simulink model "TorqueVect"  (R2022a)
settings: Solver=VariableStepAuto  StartTime=0.0  StopTime=300  RelTol=1e-3
PreLoadFcn:
  | run('Parameters\FSE_Parameters.m')
values from neighbouring files (symbols this model uses):
  Kd = 0;')    [open_carmaker_gui.m]
  Ki = 0    [open_carmaker_gui.m]
undefined symbols (not defined in the file or in its folder): BRegenEnabledButton, canChannel, CyalphaLookUp, efficiency, Fz_curve, Fz_scaling_long, gearR, izz, jw, kd, ki, Kp, kp, l_f, l_r, lambda, m, Mz_max, N, N_lat, N_long, P_max, pid_kd_lat, pid_kd_long, pid_ki_lat, pid_ki_long, pid_kp_lat, pid_kp_long, R_max, rw, steerR, T_i_max, TC_Decr_Gas, TC_Derivative, TC_Incr_Gas, TC_On, TC_Relay_Off, TC_Relay_On, tireCornerStiffness, Ts, TV_On, TV_Override, velocity_lookup, velocity_lookup_lat, y_ref, yrr_scaling
libraries: simulink x218, slpidlib x135, CarMaker4SL x73, TractionControlLibrary x13, canmsglib x9, canlib x8, TorqueVectoringLibrary x6, simulink_extras x4, PedalConversionLibrary x3, PowerControlLibrary x1
(part 10 of 26)

== system TorqueVect/CarMaker/IPG Vehicle/PowerTrain/PTControl Example/PTControl_PC_TC_MFE/New TC/TC R2 ==
  modified slip ratio reference : Inport
  lim 1 : Inport  Port=2
  modified slip ratio measurement : Inport  Port=3
  P_TC : Inport  Port=4
  D_TC : Inport  Port=5
  enable_tc : Inport  Port=6
  PID Controller : slpidlib/PID Controller  Commented=on  Controller=PD  Form=Parallel  TimeDomain=Discrete-time  UseExternalTs=off  SampleTime=-1  IntegratorMethod=Forward Euler  FilterMethod=Forward Euler  ControllerParametersSource=external  P=125  I=1  UseKiTs=on  D=0  N=100  UseFilter=on  TunerSelectOption=Transfer Function Based (PID Tuner App)  InitialConditionSource=internal  InitialConditionForIntegrator=0  InitialConditionForFilter=0  DifferentiatorICPrevScaledInput=0  ExternalReset=none  TrackingMode=off  Kt=1  LimitOutput=on  SatLimitsSource=external  UpperSaturationLimit=inf  LowerSaturationLimit=-inf  LinearizeAsGain=on  AntiWindupMode=clamping  Kb=1  POutMin=[]  POutMax=[]  IOutMin=[]  IOutMax=[]  DOutMin=[]  DOutMax=[]  NOutMin=[]  NOutMax=[]  SumOutMin=[]  SumOutMax=[]  SaturationOutMin=[]  SaturationOutMax=[]  PParamMin=[]  PParamMax=[]  IParamMin=[]  IParamMax=[]  DParamMin=[]  DParamMax=[]  NParamMin=[]  NParamMax=[]  KbParamMin=[]  KbParamMax=[]  KtParamMin=[]  KtParamMax=[]  KbOutMin=[]  KbOutMax=[]  KtOutMin=[]  KtOutMax=[]  IntegratorOutMin=[]  IntegratorOutMax=[]  FilterOutMin=[]  FilterOutMax=[]  SumI1OutMin=[]  SumI1OutMax=[]  SumI2OutMin=[]  SumI2OutMax=[]  SumI3OutMin=[]  SumI3OutMax=[]  SumI4OutMin=[]  SumI4OutMax=[]  SumDOutMin=[]  SumDOutMax=[]  DifferentiatorOutMin=[]  DifferentiatorOutMax=[]  FilterDiffOutCoefMin=[]  FilterDiffOutCoefMax=[]  ReciprocalOutMin=[]  ReciprocalOutMax=[]  SumDenOutMin=[]  SumDenOutMax=[]  SumNumOutMin=[]  SumNumOutMax=[]  DivideOutMin=[]  DivideOutMax=[]  UdiffTsProdOutMin=[]  UdiffTsProdOutMax=[]  NTsProdOutMin=[]  NTsProdOutMax=[]  UintegralTsProdOutMin=[]  UintegralTsProdOutMax=[]  UngainTsProdOutMin=[]  UngainTsProdOutMax=[]  ClampingZeroOutDataTypeStr=Inherit: Inherit via back propagation  ClampingZeroOutMin=[]  ClampingZeroOutMax=[]  FilterDenConstantOutDataTypeStr=Inherit: Inherit via back propagation  FilterDenConstantOutMin=[]  FilterDenConstantOutMax=[]  PCopyOutDataTypeStr=Inherit: Inherit via back propagation  PCopyOutMin=[]  PCopyOutMax=[]  NCopyOutDataTypeStr=Inherit: Inherit via back propagation  NCopyOutMin=[]  NCopyOutMax=[]  IntegratorContinuousStateAttributes=''  IntegratorStateMustResolveToSignalObject=off  IntegratorRTWStateStorageClass=Auto  FilterContinuousStateAttributes=''  FilterStateMustResolveToSignalObject=off  FilterRTWStateStorageClass=Auto  ParallelPVariant=ExternalParameters  IdealPVariant=Disabled  IVariant=Disabled  DVariant=ExternalParameters  IntegratorVariant=Disabled  SatVariant=External  AWVariant=Disabled  PCopyVariant=Disabled  TRVariant=Disabled  FdbkBlocksVariant=Forward  IdealPFdbkVariant=Disabled  SatFdbkVariant=Disabled  DerivativeFilterVariant=ForwardEulerFilter  NVariant=ExternalParameters  NCopyVariant=Disabled  FilterICVariant=InternalICsFilter  IntegratorICVariant=Disabled  ExternalResetVariant=Disabled  TRSumVariant=Passthrough  SumFdbkVariant=Disabled  SumVariant=Sum_PD  TsampFilterVariant=InternalTs  TsampNgainVariant=Passthrough  TsampIntegralVariant=Disabled_SignalSpec  ExternalSaturationOutDataTypeStr=Inherit: Same as second input  aMode=0
  Sum1 : Sum  Inputs=|-+
  Sum2 : Sum  Commented=on  Inputs=|-+
  traction_controller : Subsystem
  Control Effort 1 : Outport
  wires:
  modified slip ratio reference/1 -> Sum1/1
  modified slip ratio measurement/1 -> Sum1/2
  lim 1/1 -> Sum2/2, traction_controller/1(max_torque)
  PID Controller/1 -> Sum2/1
  traction_controller/1(delta_torque) -> Control Effort 1/1
  enable_tc/1 -> traction_controller/3(enable_tc)
  Sum1/1 -> traction_controller/2(dslip)
  P_TC/1 -> traction_controller/4(Kp)
  D_TC/1 -> traction_controller/5(Kd)

== system TorqueVect/CarMaker/IPG Vehicle/PowerTrain/PTControl Example/PTControl_PC_TC_MFE/New TC/TC R3 ==
  modified slip ratio reference : Inport
  lim 1 : Inport  Port=2
  modified slip ratio measurement : Inport  Port=3
  P_TC : Inport  Port=4
  D_TC : Inport  Port=5
  enable_tc : Inport  Port=6
  PID Controller : slpidlib/PID Controller  Commented=on  Controller=PD  Form=Parallel  TimeDomain=Discrete-time  UseExternalTs=off  SampleTime=-1  IntegratorMethod=Forward Euler  FilterMethod=Forward Euler  ControllerParametersSource=external  P=125  I=1  UseKiTs=on  D=0  N=100  UseFilter=on  TunerSelectOption=Transfer Function Based (PID Tuner App)  InitialConditionSource=internal  InitialConditionForIntegrator=0  InitialConditionForFilter=0  DifferentiatorICPrevScaledInput=0  ExternalReset=none  TrackingMode=off  Kt=1  LimitOutput=on  SatLimitsSource=external  UpperSaturationLimit=inf  LowerSaturationLimit=-inf  LinearizeAsGain=on  AntiWindupMode=clamping  Kb=1  POutMin=[]  POutMax=[]  IOutMin=[]  IOutMax=[]  DOutMin=[]  DOutMax=[]  NOutMin=[]  NOutMax=[]  SumOutMin=[]  SumOutMax=[]  SaturationOutMin=[]  SaturationOutMax=[]  PParamMin=[]  PParamMax=[]  IParamMin=[]  IParamMax=[]  DParamMin=[]  DParamMax=[]  NParamMin=[]  NParamMax=[]  KbParamMin=[]  KbParamMax=[]  KtParamMin=[]  KtParamMax=[]  KbOutMin=[]  KbOutMax=[]  KtOutMin=[]  KtOutMax=[]  IntegratorOutMin=[]  IntegratorOutMax=[]  FilterOutMin=[]  FilterOutMax=[]  SumI1OutMin=[]  SumI1OutMax=[]  SumI2OutMin=[]  SumI2OutMax=[]  SumI3OutMin=[]  SumI3OutMax=[]  SumI4OutMin=[]  SumI4OutMax=[]  SumDOutMin=[]  SumDOutMax=[]  DifferentiatorOutMin=[]  DifferentiatorOutMax=[]  FilterDiffOutCoefMin=[]  FilterDiffOutCoefMax=[]  ReciprocalOutMin=[]  ReciprocalOutMax=[]  SumDenOutMin=[]  SumDenOutMax=[]  SumNumOutMin=[]  SumNumOutMax=[]  DivideOutMin=[]  DivideOutMax=[]  UdiffTsProdOutMin=[]  UdiffTsProdOutMax=[]  NTsProdOutMin=[]  NTsProdOutMax=[]  UintegralTsProdOutMin=[]  UintegralTsProdOutMax=[]  UngainTsProdOutMin=[]  UngainTsProdOutMax=[]  ClampingZeroOutDataTypeStr=Inherit: Inherit via back propagation  ClampingZeroOutMin=[]  ClampingZeroOutMax=[]  FilterDenConstantOutDataTypeStr=Inherit: Inherit via back propagation  FilterDenConstantOutMin=[]  FilterDenConstantOutMax=[]  PCopyOutDataTypeStr=Inherit: Inherit via back propagation  PCopyOutMin=[]  PCopyOutMax=[]  NCopyOutDataTypeStr=Inherit: Inherit via back propagation  NCopyOutMin=[]  NCopyOutMax=[]  IntegratorContinuousStateAttributes=''  IntegratorStateMustResolveToSignalObject=off  IntegratorRTWStateStorageClass=Auto  FilterContinuousStateAttributes=''  FilterStateMustResolveToSignalObject=off  FilterRTWStateStorageClass=Auto  ParallelPVariant=ExternalParameters  IdealPVariant=Disabled  IVariant=Disabled  DVariant=ExternalParameters  IntegratorVariant=Disabled  SatVariant=External  AWVariant=Disabled  PCopyVariant=Disabled  TRVariant=Disabled  FdbkBlocksVariant=Forward  IdealPFdbkVariant=Disabled  SatFdbkVariant=Disabled  DerivativeFilterVariant=ForwardEulerFilter  NVariant=ExternalParameters  NCopyVariant=Disabled  FilterICVariant=InternalICsFilter  IntegratorICVariant=Disabled  ExternalResetVariant=Disabled  TRSumVariant=Passthrough  SumFdbkVariant=Disabled  SumVariant=Sum_PD  TsampFilterVariant=InternalTs  TsampNgainVariant=Passthrough  TsampIntegralVariant=Disabled_SignalSpec  ExternalSaturationOutDataTypeStr=Inherit: Same as second input  aMode=0
  Sum1 : Sum  Inputs=|-+
  Sum2 : Sum  Commented=on  Inputs=|-+
  traction_controller : Subsystem
  Control Effort 1 : Outport
  wires:
  modified slip ratio reference/1 -> Sum1/1
  modified slip ratio measurement/1 -> Sum1/2
  lim 1/1 -> Sum2/2, traction_controller/1(max_torque)
  PID Controller/1 -> Sum2/1
  traction_controller/1(delta_torque) -> Control Effort 1/1
  enable_tc/1 -> traction_controller/3(enable_tc)
  Sum1/1 -> traction_controller/2(dslip)
  P_TC/1 -> traction_controller/4(Kp)
  D_TC/1 -> traction_controller/5(Kd)

== system TorqueVect/CarMaker/IPG Vehicle/PowerTrain/PTControl Example/PTControl_PC_TC_MFE/New TC/TC R4 ==
  modified slip ratio reference : Inport
  lim 1 : Inport  Port=2
  modified slip ratio measurement : Inport  Port=3
  P_TC : Inport  Port=4
  D_TC : Inport  Port=5
  enable_tc : Inport  Port=6
  PID Controller : slpidlib/PID Controller  Commented=on  Controller=PD  Form=Parallel  TimeDomain=Discrete-time  UseExternalTs=off  SampleTime=-1  IntegratorMethod=Forward Euler  FilterMethod=Forward Euler  ControllerParametersSource=external  P=125  I=1  UseKiTs=on  D=0  N=100  UseFilter=on  TunerSelectOption=Transfer Function Based (PID Tuner App)  InitialConditionSource=internal  InitialConditionForIntegrator=0  InitialConditionForFilter=0  DifferentiatorICPrevScaledInput=0  ExternalReset=none  TrackingMode=off  Kt=1  LimitOutput=on  SatLimitsSource=external  UpperSaturationLimit=inf  LowerSaturationLimit=-inf  LinearizeAsGain=on  AntiWindupMode=clamping  Kb=1  POutMin=[]  POutMax=[]  IOutMin=[]  IOutMax=[]  DOutMin=[]  DOutMax=[]  NOutMin=[]  NOutMax=[]  SumOutMin=[]  SumOutMax=[]  SaturationOutMin=[]  SaturationOutMax=[]  PParamMin=[]  PParamMax=[]  IParamMin=[]  IParamMax=[]  DParamMin=[]  DParamMax=[]  NParamMin=[]  NParamMax=[]  KbParamMin=[]  KbParamMax=[]  KtParamMin=[]  KtParamMax=[]  KbOutMin=[]  KbOutMax=[]  KtOutMin=[]  KtOutMax=[]  IntegratorOutMin=[]  IntegratorOutMax=[]  FilterOutMin=[]  FilterOutMax=[]  SumI1OutMin=[]  SumI1OutMax=[]  SumI2OutMin=[]  SumI2OutMax=[]  SumI3OutMin=[]  SumI3OutMax=[]  SumI4OutMin=[]  SumI4OutMax=[]  SumDOutMin=[]  SumDOutMax=[]  DifferentiatorOutMin=[]  DifferentiatorOutMax=[]  FilterDiffOutCoefMin=[]  FilterDiffOutCoefMax=[]  ReciprocalOutMin=[]  ReciprocalOutMax=[]  SumDenOutMin=[]  SumDenOutMax=[]  SumNumOutMin=[]  SumNumOutMax=[]  DivideOutMin=[]  DivideOutMax=[]  UdiffTsProdOutMin=[]  UdiffTsProdOutMax=[]  NTsProdOutMin=[]  NTsProdOutMax=[]  UintegralTsProdOutMin=[]  UintegralTsProdOutMax=[]  UngainTsProdOutMin=[]  UngainTsProdOutMax=[]  ClampingZeroOutDataTypeStr=Inherit: Inherit via back propagation  ClampingZeroOutMin=[]  ClampingZeroOutMax=[]  FilterDenConstantOutDataTypeStr=Inherit: Inherit via back propagation  FilterDenConstantOutMin=[]  FilterDenConstantOutMax=[]  PCopyOutDataTypeStr=Inherit: Inherit via back propagation  PCopyOutMin=[]  PCopyOutMax=[]  NCopyOutDataTypeStr=Inherit: Inherit via back propagation  NCopyOutMin=[]  NCopyOutMax=[]  IntegratorContinuousStateAttributes=''  IntegratorStateMustResolveToSignalObject=off  IntegratorRTWStateStorageClass=Auto  FilterContinuousStateAttributes=''  FilterStateMustResolveToSignalObject=off  FilterRTWStateStorageClass=Auto  ParallelPVariant=ExternalParameters  IdealPVariant=Disabled  IVariant=Disabled  DVariant=ExternalParameters  IntegratorVariant=Disabled  SatVariant=External  AWVariant=Disabled  PCopyVariant=Disabled  TRVariant=Disabled  FdbkBlocksVariant=Forward  IdealPFdbkVariant=Disabled  SatFdbkVariant=Disabled  DerivativeFilterVariant=ForwardEulerFilter  NVariant=ExternalParameters  NCopyVariant=Disabled  FilterICVariant=InternalICsFilter  IntegratorICVariant=Disabled  ExternalResetVariant=Disabled  TRSumVariant=Passthrough  SumFdbkVariant=Disabled  SumVariant=Sum_PD  TsampFilterVariant=InternalTs  TsampNgainVariant=Passthrough  TsampIntegralVariant=Disabled_SignalSpec  ExternalSaturationOutDataTypeStr=Inherit: Same as second input  aMode=0
  Sum1 : Sum  Inputs=|-+
  Sum2 : Sum  Commented=on  Inputs=|-+
  traction_controller : Subsystem
  Control Effort 1 : Outport
  wires:
  modified slip ratio reference/1 -> Sum1/1
  modified slip ratio measurement/1 -> Sum1/2
  lim 1/1 -> Sum2/2, traction_controller/1(max_torque)
  PID Controller/1 -> Sum2/1
  traction_controller/1(delta_torque) -> Control Effort 1/1
  enable_tc/1 -> traction_controller/3(enable_tc)
  Sum1/1 -> traction_controller/2(dslip)
  P_TC/1 -> traction_controller/4(Kp)
  D_TC/1 -> traction_controller/5(Kd)

== system TorqueVect/CarMaker/IPG Vehicle/PowerTrain/PTControl Example/PTControl_PC_TC_MFE/Subsystem1/Subsystem ==
  rThrottlePedal : Inport
  vLong : Inport  Port=2
  BRegenEnabledButton : Inport  Port=3
  MMotorFL : Inport  Port=4
  MMotorFR : Inport  Port=5
  MMotorRL : Inport  Port=6
  MMotorRR : Inport  Port=7
  nMotorFL : Inport  Port=8
  nMotorFR : Inport  Port=9
  nMotorRL : Inport  Port=10
  nMotorRR : Inport  Port=11
  PMeasured : Inport  Port=12
  BMeasuredEnable : Inport  Port=13
  rSplitF : Inport  Port=14
  rRegenSplitF : Inport  Port=15
  PRegenLimit : Inport  Port=16
  PLimit : Inport  Port=17
  FF_PC : Inport  Port=18
  FF_RC : Inport  Port=19
  P_PC : Inport  Port=20
  D_PC : Inport  Port=21
  MMotorMax : Inport  Port=22
  Add{,1..3} (4 alike) : Sum  Inputs=-+
  PedalConversion : PedalConversionLibrary/PedalConversion  SystemSampleTime=-1  VariantActivationTime=update diagram  Latency=0  AutoFrameSizeCalculation=off
  PowerControl : PowerControlLibrary/PowerControl  SystemSampleTime=-1  VariantActivationTime=update diagram  Latency=0  AutoFrameSizeCalculation=off
  TorqueSplit : TorqueVectoringLibrary/TorqueSplit  SystemSampleTime=-1  VariantActivationTime=update diagram  Latency=0  AutoFrameSizeCalculation=off
  MMotorDemandFL : Outport
  MMotorDemandFR : Outport  Port=2
  MMotorDemandRL : Outport  Port=3
  MMotorDemandRR : Outport  Port=4
  wires:
  rThrottlePedal/1 -> [rThrottlePedal]
  [rThrottlePedal] -> PedalConversion/1
  [rThrottlePedal] -> PowerControl/13
  vLong/1 -> PedalConversion/3
  BRegenEnabledButton/1 -> PedalConversion/2
  MMotorFL/1 -> PowerControl/1
  MMotorFR/1 -> PowerControl/2
  MMotorRL/1 -> PowerControl/3
  MMotorRR/1 -> PowerControl/4
  nMotorFL/1 -> PowerControl/5
  nMotorFR/1 -> PowerControl/6
  nMotorRL/1 -> PowerControl/7
  nMotorRR/1 -> PowerControl/8
  PMeasured/1 -> PowerControl/9
  BMeasuredEnable/1 -> PowerControl/10
  PRegenLimit/1 -> PowerControl/15
  PLimit/1 -> PowerControl/16
  FF_PC/1 -> PowerControl/17
  FF_RC/1 -> PowerControl/18
  P_PC/1 -> PowerControl/19
  D_PC/1 -> PowerControl/20
  Add/1 -> MMotorDemandFL/1
  PowerControl/1 -> Add/1
  rSplitF/1 -> [rSplitF]
  [rSplitF] -> TorqueSplit/1
  rRegenSplitF/1 -> TorqueSplit/2
  PedalConversion/1 -> PowerControl/14, TorqueSplit/3
  MMotorMax/1 -> TorqueSplit/4
  [rSplitF] -> PowerControl/12
  PedalConversion/2 -> PowerControl/11
  TorqueSplit/1 -> [MMotorRequestFL]
  TorqueSplit/2 -> [MMotorRequestFR]
  TorqueSplit/3 -> [MMotorRequestRL]
  TorqueSplit/4 -> [MMotorRequestRR]
  [MMotorRequestFL] -> Add/2
  Add1/1 -> MMotorDemandFR/1
  PowerControl/2 -> Add1/1
  [MMotorRequestFR] -> Add1/2
  Add2/1 -> MMotorDemandRL/1
  PowerControl/3 -> Add2/1
  [MMotorRequestRL] -> Add2/2
  Add3/1 -> MMotorDemandRR/1
  PowerControl/4 -> Add3/1
  [MMotorRequestRR] -> Add3/2

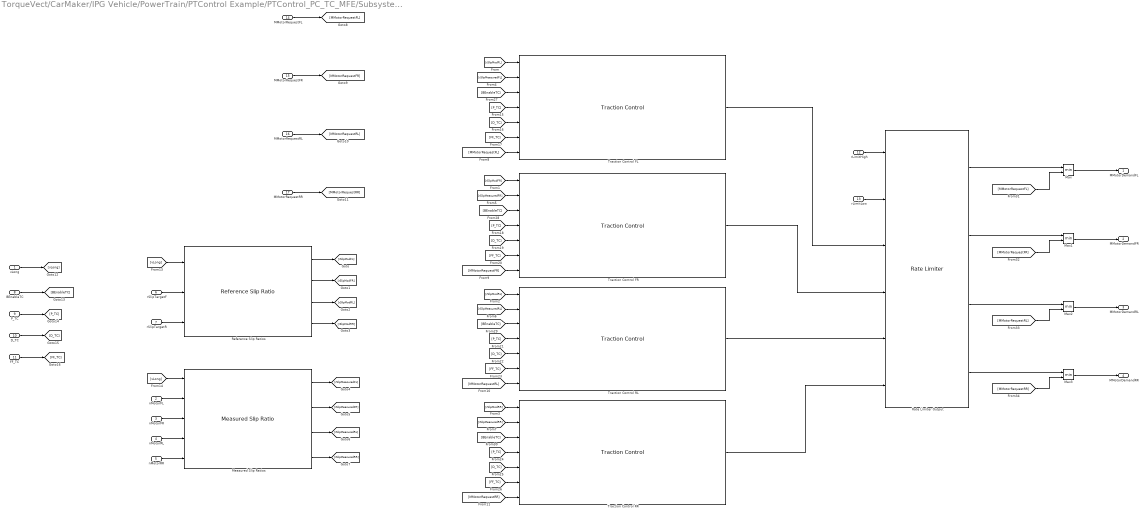
== system TorqueVect/CarMaker/IPG Vehicle/PowerTrain/PTControl Example/PTControl_PC_TC_MFE/Subsystem1/TC ==
  vLong : Inport
  nMotorFL : Inport  Port=2
  nMotorFR : Inport  Port=3
  nMotorRL : Inport  Port=4
  nMotorRR : Inport  Port=5
  rSlipTargetF : Inport  Port=6
  rSlipTargetR : Inport  Port=7
  BEnableTC : Inport  Port=8
  P_TC : Inport  Port=9
  D_TC : Inport  Port=10
  FF_TC : Inport  Port=11
  rLimitHigh : Inport  Port=12
  rLimitLow : Inport  Port=13
  MMotorRequestFL : Inport  Port=14
  MMotorRequestFR : Inport  Port=15
  MMotorRequestRL : Inport  Port=16
  MMotorRequestRR : Inport  Port=17
  Max{,1..3} (4 alike) : MinMax  Inputs=2
  Measured Slip Ratios : TractionControlLibrary/Measured Slip Ratio  SystemSampleTime=-1  VariantActivationTime=update diagram  Latency=0  AutoFrameSizeCalculation=off
  Rate Limiter Output : TractionControlLibrary/Rate Limiter  SystemSampleTime=-1  VariantActivationTime=update diagram  Latency=0  AutoFrameSizeCalculation=off
  Reference Slip Ratios : TractionControlLibrary/Reference Slip Ratio  SystemSampleTime=-1  VariantActivationTime=update diagram  Latency=0  AutoFrameSizeCalculation=off
  Traction Control FL : TractionControlLibrary/Traction Control  SystemSampleTime=-1  VariantActivationTime=update diagram  Latency=0  AutoFrameSizeCalculation=off
  Traction Control FR : TractionControlLibrary/Traction Control  SystemSampleTime=-1  VariantActivationTime=update diagram  Latency=0  AutoFrameSizeCalculation=off
  Traction Control RL : TractionControlLibrary/Traction Control  SystemSampleTime=-1  VariantActivationTime=update diagram  Latency=0  AutoFrameSizeCalculation=off
  Traction Control RR : TractionControlLibrary/Traction Control  SystemSampleTime=-1  VariantActivationTime=update diagram  Latency=0  AutoFrameSizeCalculation=off
  MMotorDemandFL : Outport
  MMotorDemandFR : Outport  Port=2
  MMotorDemandRL : Outport  Port=3
  MMotorDemandRR : Outport  Port=4
  wires:
  Traction Control FL/1 -> Rate Limiter Output/3
  Traction Control FR/1 -> Rate Limiter Output/4
  Traction Control RL/1 -> Rate Limiter Output/5
  Traction Control RR/1 -> Rate Limiter Output/6
  Reference Slip Ratios/1 -> [rSlipModFL]
  Reference Slip Ratios/2 -> [rSlipModFR]
  Reference Slip Ratios/3 -> [rSlipModRL]
  Reference Slip Ratios/4 -> [rSlipModRR]
  [rSlipModFL] -> Traction Control FL/1
  [rSlipModFR] -> Traction Control FR/1
  [rSlipModRL] -> Traction Control RL/1
  [rSlipModRR] -> Traction Control RR/1
  Measured Slip Ratios/1 -> [rSlipMeasuredFL]
  Measured Slip Ratios/2 -> [rSlipMeasuredFR]
  Measured Slip Ratios/3 -> [rSlipMeasuredRL]
  Measured Slip Ratios/4 -> [rSlipMeasuredRR]
  [rSlipMeasuredFL] -> Traction Control FL/2
  [rSlipMeasuredFR] -> Traction Control FR/2
  [rSlipMeasuredRL] -> Traction Control RL/2
  [rSlipMeasuredRR] -> Traction Control RR/2
  MMotorRequestFL/1 -> [MMotorRequestFL]
  MMotorRequestFR/1 -> [MMotorRequestFR]
  MMotorRequestRL/1 -> [MMotorRequestRL]
  MMotorRequestRR/1 -> [MMotorRequestRR]
  [MMotorRequestFL] -> Traction Control FL/7
  [MMotorRequestFR] -> Traction Control FR/7
  [MMotorRequestRL] -> Traction Control RL/7
  [MMotorRequestRR] -> Traction Control RR/7
  vLong/1 -> [vLong]
  [vLong] -> Reference Slip Ratios/1
  [vLong] -> Measured Slip Ratios/1
  nMotorFL/1 -> Measured Slip Ratios/2
  nMotorFR/1 -> Measured Slip Ratios/3
  nMotorRL/1 -> Measured Slip Ratios/4
  nMotorRR/1 -> Measured Slip Ratios/5
  rSlipTargetF/1 -> Reference Slip Ratios/2
  rSlipTargetR/1 -> Reference Slip Ratios/3
  BEnableTC/1 -> [BEnableTC]
  P_TC/1 -> [P_TC]
  D_TC/1 -> [D_TC]
  FF_TC/1 -> [FF_TC]
  [P_TC] -> Traction Control FL/4
  [D_TC] -> Traction Control FL/5
  [FF_TC] -> Traction Control FL/6
  [FF_TC] -> Traction Control FR/6
  [D_TC] -> Traction Control FR/5
  [P_TC] -> Traction Control FR/4
  [FF_TC] -> Traction Control RL/6
  [D_TC] -> Traction Control RL/5
  [P_TC] -> Traction Control RL/4
  [FF_TC] -> Traction Control RR/6
  [D_TC] -> Traction Control RR/5
  [P_TC] -> Traction Control RR/4
  [BEnableTC] -> Traction Control FL/3
  [BEnableTC] -> Traction Control FR/3
  [BEnableTC] -> Traction Control RL/3
  [BEnableTC] -> Traction Control RR/3
  rLimitHigh/1 -> Rate Limiter Output/1
  rLimitLow/1 -> Rate Limiter Output/2
  Rate Limiter Output/1 -> Max/1
  [MMotorRequestFL] -> Max/2
  Max/1 -> MMotorDemandFL/1
  Rate Limiter Output/2 -> Max1/1
  Max1/1 -> MMotorDemandFR/1
  [MMotorRequestFR] -> Max1/2
  Rate Limiter Output/3 -> Max2/1
  Max2/1 -> MMotorDemandRL/1
  [MMotorRequestRL] -> Max2/2
  Rate Limiter Output/4 -> Max3/1
  Max3/1 -> MMotorDemandRR/1
  [MMotorRequestRR] -> Max3/2

== system TorqueVect/CarMaker/IPG Vehicle/PowerTrain/PTControl Example/PTControl_TC_MFE/New TC/Reference Generator1 ==
  note: Modified slip ratio targets
  note: Vehicle velocity
  note: For throttle sign and Product:
      | If positive, normal reference
      | If negative (regen), similar reference but negative (negative target slip*times speed), this might need to change to account for regen limits
      | If 0, target zero
  x2 : Inport
  Front SR Target : Inport  Port=2
  Rear SR Target : Inport  Port=3
  Constant : Constant
  Product1 : Product
  Product2 : Product
  Switch : Switch  Criteria=u2 > Threshold  Threshold=1  SaturateOnIntegerOverflow=off  InputSameDT=off
  R1 : Outport
  L1 : Outport  Port=2
  R2 : Outport  Port=3
  L2 : Outport  Port=4
  wires:
  Front SR Target/1 -> Product1/1
  Product1/1 -> L1/1, R1/1
  Product2/1 -> L2/1, R2/1
  Rear SR Target/1 -> Product2/2
  Switch/1 -> Product2/1, Product1/2
  x2/1 -> Switch/1, Switch/2
  Constant/1 -> Switch/3

== system TorqueVect/CarMaker/IPG Vehicle/PowerTrain/PTControl Example/PTControl_TC_MFE/New TC/TC R1 ==
  modified slip ratio reference : Inport
  lim 1 : Inport  Port=2
  modified slip ratio measurement : Inport  Port=3
  P_TC : Inport  Port=4
  D_TC : Inport  Port=5
  enable_tc : Inport  Port=6
  PID Controller : slpidlib/PID Controller  Commented=on  Controller=PD  Form=Parallel  TimeDomain=Discrete-time  UseExternalTs=off  SampleTime=-1  IntegratorMethod=Forward Euler  FilterMethod=Forward Euler  ControllerParametersSource=external  P=125  I=1  UseKiTs=on  D=0  N=100  UseFilter=on  TunerSelectOption=Transfer Function Based (PID Tuner App)  InitialConditionSource=internal  InitialConditionForIntegrator=0  InitialConditionForFilter=0  DifferentiatorICPrevScaledInput=0  ExternalReset=none  TrackingMode=off  Kt=1  LimitOutput=on  SatLimitsSource=external  UpperSaturationLimit=inf  LowerSaturationLimit=-inf  LinearizeAsGain=on  AntiWindupMode=clamping  Kb=1  POutMin=[]  POutMax=[]  IOutMin=[]  IOutMax=[]  DOutMin=[]  DOutMax=[]  NOutMin=[]  NOutMax=[]  SumOutMin=[]  SumOutMax=[]  SaturationOutMin=[]  SaturationOutMax=[]  PParamMin=[]  PParamMax=[]  IParamMin=[]  IParamMax=[]  DParamMin=[]  DParamMax=[]  NParamMin=[]  NParamMax=[]  KbParamMin=[]  KbParamMax=[]  KtParamMin=[]  KtParamMax=[]  KbOutMin=[]  KbOutMax=[]  KtOutMin=[]  KtOutMax=[]  IntegratorOutMin=[]  IntegratorOutMax=[]  FilterOutMin=[]  FilterOutMax=[]  SumI1OutMin=[]  SumI1OutMax=[]  SumI2OutMin=[]  SumI2OutMax=[]  SumI3OutMin=[]  SumI3OutMax=[]  SumI4OutMin=[]  SumI4OutMax=[]  SumDOutMin=[]  SumDOutMax=[]  DifferentiatorOutMin=[]  DifferentiatorOutMax=[]  FilterDiffOutCoefMin=[]  FilterDiffOutCoefMax=[]  ReciprocalOutMin=[]  ReciprocalOutMax=[]  SumDenOutMin=[]  SumDenOutMax=[]  SumNumOutMin=[]  SumNumOutMax=[]  DivideOutMin=[]  DivideOutMax=[]  UdiffTsProdOutMin=[]  UdiffTsProdOutMax=[]  NTsProdOutMin=[]  NTsProdOutMax=[]  UintegralTsProdOutMin=[]  UintegralTsProdOutMax=[]  UngainTsProdOutMin=[]  UngainTsProdOutMax=[]  ClampingZeroOutDataTypeStr=Inherit: Inherit via back propagation  ClampingZeroOutMin=[]  ClampingZeroOutMax=[]  FilterDenConstantOutDataTypeStr=Inherit: Inherit via back propagation  FilterDenConstantOutMin=[]  FilterDenConstantOutMax=[]  PCopyOutDataTypeStr=Inherit: Inherit via back propagation  PCopyOutMin=[]  PCopyOutMax=[]  NCopyOutDataTypeStr=Inherit: Inherit via back propagation  NCopyOutMin=[]  NCopyOutMax=[]  IntegratorContinuousStateAttributes=''  IntegratorStateMustResolveToSignalObject=off  IntegratorRTWStateStorageClass=Auto  FilterContinuousStateAttributes=''  FilterStateMustResolveToSignalObject=off  FilterRTWStateStorageClass=Auto  ParallelPVariant=ExternalParameters  IdealPVariant=Disabled  IVariant=Disabled  DVariant=ExternalParameters  IntegratorVariant=Disabled  SatVariant=External  AWVariant=Disabled  PCopyVariant=Disabled  TRVariant=Disabled  FdbkBlocksVariant=Forward  IdealPFdbkVariant=Disabled  SatFdbkVariant=Disabled  DerivativeFilterVariant=ForwardEulerFilter  NVariant=ExternalParameters  NCopyVariant=Disabled  FilterICVariant=InternalICsFilter  IntegratorICVariant=Disabled  ExternalResetVariant=Disabled  TRSumVariant=Passthrough  SumFdbkVariant=Disabled  SumVariant=Sum_PD  TsampFilterVariant=InternalTs  TsampNgainVariant=Passthrough  TsampIntegralVariant=Disabled_SignalSpec  ExternalSaturationOutDataTypeStr=Inherit: Same as second input  aMode=0
  Sum1 : Sum  Inputs=|-+
  Sum2 : Sum  Commented=on  Inputs=|-+
  traction_controller : Subsystem
  Control Effort 1 : Outport
  wires:
  modified slip ratio reference/1 -> Sum1/1
  modified slip ratio measurement/1 -> Sum1/2
  lim 1/1 -> Sum2/2, traction_controller/1(max_torque)
  PID Controller/1 -> Sum2/1
  traction_controller/1(delta_torque) -> Control Effort 1/1
  enable_tc/1 -> traction_controller/3(enable_tc)
  Sum1/1 -> traction_controller/2(dslip)
  P_TC/1 -> traction_controller/4(Kp)
  D_TC/1 -> traction_controller/5(Kd)

== system TorqueVect/CarMaker/IPG Vehicle/PowerTrain/PTControl Example/PTControl_TC_MFE/New TC/TC R2 ==
  modified slip ratio reference : Inport
  lim 1 : Inport  Port=2
  modified slip ratio measurement : Inport  Port=3
  P_TC : Inport  Port=4
  D_TC : Inport  Port=5
  enable_tc : Inport  Port=6
  PID Controller : slpidlib/PID Controller  Commented=on  Controller=PD  Form=Parallel  TimeDomain=Discrete-time  UseExternalTs=off  SampleTime=-1  IntegratorMethod=Forward Euler  FilterMethod=Forward Euler  ControllerParametersSource=external  P=125  I=1  UseKiTs=on  D=0  N=100  UseFilter=on  TunerSelectOption=Transfer Function Based (PID Tuner App)  InitialConditionSource=internal  InitialConditionForIntegrator=0  InitialConditionForFilter=0  DifferentiatorICPrevScaledInput=0  ExternalReset=none  TrackingMode=off  Kt=1  LimitOutput=on  SatLimitsSource=external  UpperSaturationLimit=inf  LowerSaturationLimit=-inf  LinearizeAsGain=on  AntiWindupMode=clamping  Kb=1  POutMin=[]  POutMax=[]  IOutMin=[]  IOutMax=[]  DOutMin=[]  DOutMax=[]  NOutMin=[]  NOutMax=[]  SumOutMin=[]  SumOutMax=[]  SaturationOutMin=[]  SaturationOutMax=[]  PParamMin=[]  PParamMax=[]  IParamMin=[]  IParamMax=[]  DParamMin=[]  DParamMax=[]  NParamMin=[]  NParamMax=[]  KbParamMin=[]  KbParamMax=[]  KtParamMin=[]  KtParamMax=[]  KbOutMin=[]  KbOutMax=[]  KtOutMin=[]  KtOutMax=[]  IntegratorOutMin=[]  IntegratorOutMax=[]  FilterOutMin=[]  FilterOutMax=[]  SumI1OutMin=[]  SumI1OutMax=[]  SumI2OutMin=[]  SumI2OutMax=[]  SumI3OutMin=[]  SumI3OutMax=[]  SumI4OutMin=[]  SumI4OutMax=[]  SumDOutMin=[]  SumDOutMax=[]  DifferentiatorOutMin=[]  DifferentiatorOutMax=[]  FilterDiffOutCoefMin=[]  FilterDiffOutCoefMax=[]  ReciprocalOutMin=[]  ReciprocalOutMax=[]  SumDenOutMin=[]  SumDenOutMax=[]  SumNumOutMin=[]  SumNumOutMax=[]  DivideOutMin=[]  DivideOutMax=[]  UdiffTsProdOutMin=[]  UdiffTsProdOutMax=[]  NTsProdOutMin=[]  NTsProdOutMax=[]  UintegralTsProdOutMin=[]  UintegralTsProdOutMax=[]  UngainTsProdOutMin=[]  UngainTsProdOutMax=[]  ClampingZeroOutDataTypeStr=Inherit: Inherit via back propagation  ClampingZeroOutMin=[]  ClampingZeroOutMax=[]  FilterDenConstantOutDataTypeStr=Inherit: Inherit via back propagation  FilterDenConstantOutMin=[]  FilterDenConstantOutMax=[]  PCopyOutDataTypeStr=Inherit: Inherit via back propagation  PCopyOutMin=[]  PCopyOutMax=[]  NCopyOutDataTypeStr=Inherit: Inherit via back propagation  NCopyOutMin=[]  NCopyOutMax=[]  IntegratorContinuousStateAttributes=''  IntegratorStateMustResolveToSignalObject=off  IntegratorRTWStateStorageClass=Auto  FilterContinuousStateAttributes=''  FilterStateMustResolveToSignalObject=off  FilterRTWStateStorageClass=Auto  ParallelPVariant=ExternalParameters  IdealPVariant=Disabled  IVariant=Disabled  DVariant=ExternalParameters  IntegratorVariant=Disabled  SatVariant=External  AWVariant=Disabled  PCopyVariant=Disabled  TRVariant=Disabled  FdbkBlocksVariant=Forward  IdealPFdbkVariant=Disabled  SatFdbkVariant=Disabled  DerivativeFilterVariant=ForwardEulerFilter  NVariant=ExternalParameters  NCopyVariant=Disabled  FilterICVariant=InternalICsFilter  IntegratorICVariant=Disabled  ExternalResetVariant=Disabled  TRSumVariant=Passthrough  SumFdbkVariant=Disabled  SumVariant=Sum_PD  TsampFilterVariant=InternalTs  TsampNgainVariant=Passthrough  TsampIntegralVariant=Disabled_SignalSpec  ExternalSaturationOutDataTypeStr=Inherit: Same as second input  aMode=0
  Sum1 : Sum  Inputs=|-+
  Sum2 : Sum  Commented=on  Inputs=|-+
  traction_controller : Subsystem
  Control Effort 1 : Outport
  wires:
  modified slip ratio reference/1 -> Sum1/1
  modified slip ratio measurement/1 -> Sum1/2
  lim 1/1 -> Sum2/2, traction_controller/1(max_torque)
  PID Controller/1 -> Sum2/1
  traction_controller/1(delta_torque) -> Control Effort 1/1
  enable_tc/1 -> traction_controller/3(enable_tc)
  Sum1/1 -> traction_controller/2(dslip)
  P_TC/1 -> traction_controller/4(Kp)
  D_TC/1 -> traction_controller/5(Kd)

== system TorqueVect/CarMaker/IPG Vehicle/PowerTrain/PTControl Example/PTControl_TC_MFE/New TC/TC R3 ==
  modified slip ratio reference : Inport
  lim 1 : Inport  Port=2
  modified slip ratio measurement : Inport  Port=3
  P_TC : Inport  Port=4
  D_TC : Inport  Port=5
  enable_tc : Inport  Port=6
  PID Controller : slpidlib/PID Controller  Commented=on  Controller=PD  Form=Parallel  TimeDomain=Discrete-time  UseExternalTs=off  SampleTime=-1  IntegratorMethod=Forward Euler  FilterMethod=Forward Euler  ControllerParametersSource=external  P=125  I=1  UseKiTs=on  D=0  N=100  UseFilter=on  TunerSelectOption=Transfer Function Based (PID Tuner App)  InitialConditionSource=internal  InitialConditionForIntegrator=0  InitialConditionForFilter=0  DifferentiatorICPrevScaledInput=0  ExternalReset=none  TrackingMode=off  Kt=1  LimitOutput=on  SatLimitsSource=external  UpperSaturationLimit=inf  LowerSaturationLimit=-inf  LinearizeAsGain=on  AntiWindupMode=clamping  Kb=1  POutMin=[]  POutMax=[]  IOutMin=[]  IOutMax=[]  DOutMin=[]  DOutMax=[]  NOutMin=[]  NOutMax=[]  SumOutMin=[]  SumOutMax=[]  SaturationOutMin=[]  SaturationOutMax=[]  PParamMin=[]  PParamMax=[]  IParamMin=[]  IParamMax=[]  DParamMin=[]  DParamMax=[]  NParamMin=[]  NParamMax=[]  KbParamMin=[]  KbParamMax=[]  KtParamMin=[]  KtParamMax=[]  KbOutMin=[]  KbOutMax=[]  KtOutMin=[]  KtOutMax=[]  IntegratorOutMin=[]  IntegratorOutMax=[]  FilterOutMin=[]  FilterOutMax=[]  SumI1OutMin=[]  SumI1OutMax=[]  SumI2OutMin=[]  SumI2OutMax=[]  SumI3OutMin=[]  SumI3OutMax=[]  SumI4OutMin=[]  SumI4OutMax=[]  SumDOutMin=[]  SumDOutMax=[]  DifferentiatorOutMin=[]  DifferentiatorOutMax=[]  FilterDiffOutCoefMin=[]  FilterDiffOutCoefMax=[]  ReciprocalOutMin=[]  ReciprocalOutMax=[]  SumDenOutMin=[]  SumDenOutMax=[]  SumNumOutMin=[]  SumNumOutMax=[]  DivideOutMin=[]  DivideOutMax=[]  UdiffTsProdOutMin=[]  UdiffTsProdOutMax=[]  NTsProdOutMin=[]  NTsProdOutMax=[]  UintegralTsProdOutMin=[]  UintegralTsProdOutMax=[]  UngainTsProdOutMin=[]  UngainTsProdOutMax=[]  ClampingZeroOutDataTypeStr=Inherit: Inherit via back propagation  ClampingZeroOutMin=[]  ClampingZeroOutMax=[]  FilterDenConstantOutDataTypeStr=Inherit: Inherit via back propagation  FilterDenConstantOutMin=[]  FilterDenConstantOutMax=[]  PCopyOutDataTypeStr=Inherit: Inherit via back propagation  PCopyOutMin=[]  PCopyOutMax=[]  NCopyOutDataTypeStr=Inherit: Inherit via back propagation  NCopyOutMin=[]  NCopyOutMax=[]  IntegratorContinuousStateAttributes=''  IntegratorStateMustResolveToSignalObject=off  IntegratorRTWStateStorageClass=Auto  FilterContinuousStateAttributes=''  FilterStateMustResolveToSignalObject=off  FilterRTWStateStorageClass=Auto  ParallelPVariant=ExternalParameters  IdealPVariant=Disabled  IVariant=Disabled  DVariant=ExternalParameters  IntegratorVariant=Disabled  SatVariant=External  AWVariant=Disabled  PCopyVariant=Disabled  TRVariant=Disabled  FdbkBlocksVariant=Forward  IdealPFdbkVariant=Disabled  SatFdbkVariant=Disabled  DerivativeFilterVariant=ForwardEulerFilter  NVariant=ExternalParameters  NCopyVariant=Disabled  FilterICVariant=InternalICsFilter  IntegratorICVariant=Disabled  ExternalResetVariant=Disabled  TRSumVariant=Passthrough  SumFdbkVariant=Disabled  SumVariant=Sum_PD  TsampFilterVariant=InternalTs  TsampNgainVariant=Passthrough  TsampIntegralVariant=Disabled_SignalSpec  ExternalSaturationOutDataTypeStr=Inherit: Same as second input  aMode=0
  Sum1 : Sum  Inputs=|-+
  Sum2 : Sum  Commented=on  Inputs=|-+
  traction_controller : Subsystem
  Control Effort 1 : Outport
  wires:
  modified slip ratio reference/1 -> Sum1/1
  modified slip ratio measurement/1 -> Sum1/2
  lim 1/1 -> Sum2/2, traction_controller/1(max_torque)
  PID Controller/1 -> Sum2/1
  traction_controller/1(delta_torque) -> Control Effort 1/1
  enable_tc/1 -> traction_controller/3(enable_tc)
  Sum1/1 -> traction_controller/2(dslip)
  P_TC/1 -> traction_controller/4(Kp)
  D_TC/1 -> traction_controller/5(Kd)

== system TorqueVect/CarMaker/IPG Vehicle/PowerTrain/PTControl Example/PTControl_TC_MFE/New TC/TC R4 ==
  modified slip ratio reference : Inport
  lim 1 : Inport  Port=2
  modified slip ratio measurement : Inport  Port=3
  P_TC : Inport  Port=4
  D_TC : Inport  Port=5
  enable_tc : Inport  Port=6
  PID Controller : slpidlib/PID Controller  Commented=on  Controller=PD  Form=Parallel  TimeDomain=Discrete-time  UseExternalTs=off  SampleTime=-1  IntegratorMethod=Forward Euler  FilterMethod=Forward Euler  ControllerParametersSource=external  P=125  I=1  UseKiTs=on  D=0  N=100  UseFilter=on  TunerSelectOption=Transfer Function Based (PID Tuner App)  InitialConditionSource=internal  InitialConditionForIntegrator=0  InitialConditionForFilter=0  DifferentiatorICPrevScaledInput=0  ExternalReset=none  TrackingMode=off  Kt=1  LimitOutput=on  SatLimitsSource=external  UpperSaturationLimit=inf  LowerSaturationLimit=-inf  LinearizeAsGain=on  AntiWindupMode=clamping  Kb=1  POutMin=[]  POutMax=[]  IOutMin=[]  IOutMax=[]  DOutMin=[]  DOutMax=[]  NOutMin=[]  NOutMax=[]  SumOutMin=[]  SumOutMax=[]  SaturationOutMin=[]  SaturationOutMax=[]  PParamMin=[]  PParamMax=[]  IParamMin=[]  IParamMax=[]  DParamMin=[]  DParamMax=[]  NParamMin=[]  NParamMax=[]  KbParamMin=[]  KbParamMax=[]  KtParamMin=[]  KtParamMax=[]  KbOutMin=[]  KbOutMax=[]  KtOutMin=[]  KtOutMax=[]  IntegratorOutMin=[]  IntegratorOutMax=[]  FilterOutMin=[]  FilterOutMax=[]  SumI1OutMin=[]  SumI1OutMax=[]  SumI2OutMin=[]  SumI2OutMax=[]  SumI3OutMin=[]  SumI3OutMax=[]  SumI4OutMin=[]  SumI4OutMax=[]  SumDOutMin=[]  SumDOutMax=[]  DifferentiatorOutMin=[]  DifferentiatorOutMax=[]  FilterDiffOutCoefMin=[]  FilterDiffOutCoefMax=[]  ReciprocalOutMin=[]  ReciprocalOutMax=[]  SumDenOutMin=[]  SumDenOutMax=[]  SumNumOutMin=[]  SumNumOutMax=[]  DivideOutMin=[]  DivideOutMax=[]  UdiffTsProdOutMin=[]  UdiffTsProdOutMax=[]  NTsProdOutMin=[]  NTsProdOutMax=[]  UintegralTsProdOutMin=[]  UintegralTsProdOutMax=[]  UngainTsProdOutMin=[]  UngainTsProdOutMax=[]  ClampingZeroOutDataTypeStr=Inherit: Inherit via back propagation  ClampingZeroOutMin=[]  ClampingZeroOutMax=[]  FilterDenConstantOutDataTypeStr=Inherit: Inherit via back propagation  FilterDenConstantOutMin=[]  FilterDenConstantOutMax=[]  PCopyOutDataTypeStr=Inherit: Inherit via back propagation  PCopyOutMin=[]  PCopyOutMax=[]  NCopyOutDataTypeStr=Inherit: Inherit via back propagation  NCopyOutMin=[]  NCopyOutMax=[]  IntegratorContinuousStateAttributes=''  IntegratorStateMustResolveToSignalObject=off  IntegratorRTWStateStorageClass=Auto  FilterContinuousStateAttributes=''  FilterStateMustResolveToSignalObject=off  FilterRTWStateStorageClass=Auto  ParallelPVariant=ExternalParameters  IdealPVariant=Disabled  IVariant=Disabled  DVariant=ExternalParameters  IntegratorVariant=Disabled  SatVariant=External  AWVariant=Disabled  PCopyVariant=Disabled  TRVariant=Disabled  FdbkBlocksVariant=Forward  IdealPFdbkVariant=Disabled  SatFdbkVariant=Disabled  DerivativeFilterVariant=ForwardEulerFilter  NVariant=ExternalParameters  NCopyVariant=Disabled  FilterICVariant=InternalICsFilter  IntegratorICVariant=Disabled  ExternalResetVariant=Disabled  TRSumVariant=Passthrough  SumFdbkVariant=Disabled  SumVariant=Sum_PD  TsampFilterVariant=InternalTs  TsampNgainVariant=Passthrough  TsampIntegralVariant=Disabled_SignalSpec  ExternalSaturationOutDataTypeStr=Inherit: Same as second input  aMode=0
  Sum1 : Sum  Inputs=|-+
  Sum2 : Sum  Commented=on  Inputs=|-+
  traction_controller : Subsystem
  Control Effort 1 : Outport
  wires:
  modified slip ratio reference/1 -> Sum1/1
  modified slip ratio measurement/1 -> Sum1/2
  lim 1/1 -> Sum2/2, traction_controller/1(max_torque)
  PID Controller/1 -> Sum2/1
  traction_controller/1(delta_torque) -> Control Effort 1/1
  enable_tc/1 -> traction_controller/3(enable_tc)
  Sum1/1 -> traction_controller/2(dslip)
  P_TC/1 -> traction_controller/4(Kp)
  D_TC/1 -> traction_controller/5(Kd)

== system TorqueVect/CarMaker/IPG Vehicle/PowerTrain/PTControl Example/PTControl_TC_MFE/TC/Rate Limiter Output ==
  rLimitHigh : Inport
  rLimitLow : Inport  Port=2
  MMotorDemandedFL : Inport  Port=3
  MMotorDemandedFR : Inport  Port=4
  MMotorDemandedRL : Inport  Port=5
  MMotorDemandedRR : Inport  Port=6
  Rate Limiter{,1..3} (4 alike) : RateLimiter  RisingSlewLimit=50  FallingSlewLimit=-50  SampleTimeMode=inherited
  Terminator : Terminator
  Terminator1 : Terminator
  MMotorDemandFL : Outport
  MMotorDemandFR : Outport  Port=2
  MMotorDemandRL : Outport  Port=3
  MMotorDemandRR : Outport  Port=4
  wires:
  MMotorDemandedRR/1 -> Rate Limiter3/1
  MMotorDemandedRL/1 -> Rate Limiter2/1
  MMotorDemandedFR/1 -> Rate Limiter1/1
  MMotorDemandedFL/1 -> Rate Limiter/1
  Rate Limiter3/1 -> MMotorDemandRR/1
  Rate Limiter2/1 -> MMotorDemandRL/1
  Rate Limiter1/1 -> MMotorDemandFR/1
  Rate Limiter/1 -> MMotorDemandFL/1
  rLimitHigh/1 -> Terminator/1
  rLimitLow/1 -> Terminator1/1

== system TorqueVect/CarMaker/IPG Vehicle/PowerTrain/PTControl Example/PTControl_TV_IPG/Torque Control 0/Electronic Gas Pedal FL ==
  TV_On : Inport
  VC.Gas : Inport  Port=2
  Define CM Dict : CarMaker4SL/Define CM Dict  xname=E_Gas_FL  xmono=off  xtype=Double4  xdvaplace=None  xnstates=0  xfirststate=0  xinitial=0
  Read CM Dict : CarMaker4SL/Read CM Dict  xname=E_Gas_FL  xsync=off  xstime=Continuous
  Read CM Dict1 : CarMaker4SL/Read CM Dict  xname=Car.LongSlipFL  xsync=off  xstime=Continuous
  Switch : Switch  Criteria=u2 > Threshold  SaturateOnIntegerOverflow=off  InputSameDT=off
  Traction Control FL : Subsystem
  Write CM Dict : CarMaker4SL/Write CM Dict  xname=E_Gas_FL  xsync=off
  Motor_Gas_FL : Outport  VectorParamsAs1DForOutWhenUnconnected=off
  wires:
  Read CM Dict/1 -> Traction Control FL/2(E_Gas.)
  Read CM Dict1/1 -> Traction Control FL/3(Car.LongSlip)
  VC.Gas/1 -> Switch/3, Traction Control FL/1(VC.Gas)
  Switch/1 -> Motor_Gas_FL/1
  TV_On/1 -> Switch/2
  Traction Control FL/1(E_Gas) -> Switch/1, Write CM Dict/1

== system TorqueVect/CarMaker/IPG Vehicle/PowerTrain/PTControl Example/PTControl_TV_IPG/Torque Control 0/Torque Vectoring FL ==
  Abs : Abs  SaturateOnIntegerOverflow=off
  Abs2 : Abs  SaturateOnIntegerOverflow=off
  Constant : Constant
  Divide : Product  Inputs=*/
  Gain : Gain  Gain=-1
  Gravity : Gain  Gain=9.81
  Lookup Table : Lookup  InputValues=[0,0.1,0.2,0.3,0.4,0.5,0.6,0.7,0.8,1,2,3,4]  Table=[0,0,0.05,0.1,0.2,0.3,0.4,0.5,0.6,0.7,1,1,1]  SaturateOnIntegerOverflow=off
  Override : Gain  Gain=TV_Override
  Product : Product  RndMeth=Zero
  Read CM Dict : CarMaker4SL/Read CM Dict  xname=Car.muRoadFL  xsync=off  xstime=Continuous
  Read CM Dict1 : CarMaker4SL/Read CM Dict  xname=Car.v  xsync=off  xstime=Continuous
  Read CM Dict2 : CarMaker4SL/Read CM Dict  xname=Car.YawRate  xsync=off  xstime=Continuous
  Read CM Dict3 : CarMaker4SL/Read CM Dict  xname=VC.Steer.Ang  xsync=off  xstime=Continuous
  Subtract : Sum  Inputs=+-
  Switch : Switch  Criteria=u2 > Threshold  SaturateOnIntegerOverflow=off  InputSameDT=off
  TV FL : Outport  VectorParamsAs1DForOutWhenUnconnected=off
  wires:
  Gain/1 -> Lookup Table/1
  Abs2/1 -> Subtract/2
  Lookup Table/1 -> Product/2
  Read CM Dict3/1 -> Gain/1
  Product/1 -> TV FL/1
  Subtract/1 -> Product/1
  Read CM Dict2/1 -> Abs2/1
  Divide/1 -> Subtract/1
  Abs/1 -> Divide/2
  Switch/1 -> Abs/1
  Constant/1 -> Switch/3
  Read CM Dict1/1 -> Switch/2, Switch/1
  Override/1 -> Divide/1
  Gravity/1 -> Override/1
  Read CM Dict/1 -> Gravity/1

== system TorqueVect/CarMaker/IPG Vehicle/PowerTrain/PTControl Example/PTControl_TV_IPG/Torque Control 1/Electronic Gas Pedal FR ==
  TV_On : Inport
  VC.Gas : Inport  Port=2
  Define CM Dict : CarMaker4SL/Define CM Dict  xname=E_Gas_FR  xmono=off  xtype=Double4  xdvaplace=None  xnstates=0  xfirststate=0  xinitial=0
  Read CM Dict : CarMaker4SL/Read CM Dict  xname=E_Gas_FR  xsync=off  xstime=Continuous
  Read CM Dict1 : CarMaker4SL/Read CM Dict  xname=Car.LongSlipFR  xsync=off  xstime=Continuous
  Switch : Switch  Criteria=u2 > Threshold  SaturateOnIntegerOverflow=off  InputSameDT=off
  Traction Control FR : Subsystem
  Write CM Dict : CarMaker4SL/Write CM Dict  xname=E_Gas_FR  xsync=off
  Motor_Gas_FR : Outport  VectorParamsAs1DForOutWhenUnconnected=off
  wires:
  Traction Control FR/1(E_Gas) -> Write CM Dict/1, Switch/1
  TV_On/1 -> Switch/2
  Switch/1 -> Motor_Gas_FR/1
  VC.Gas/1 -> Traction Control FR/1(VC.Gas), Switch/3
  Read CM Dict1/1 -> Traction Control FR/3(Car.LongSlip)
  Read CM Dict/1 -> Traction Control FR/2(E_Gas.)

== system TorqueVect/CarMaker/IPG Vehicle/PowerTrain/PTControl Example/PTControl_TV_IPG/Torque Control 1/Torque Vectoring FR ==
  Abs : Abs  SaturateOnIntegerOverflow=off
  Abs2 : Abs  SaturateOnIntegerOverflow=off
  Constant : Constant
  Divide : Product  Inputs=*/
  Gain : Gain  Gain=-1
  Gravity : Gain  Gain=9.81
  Lookup Table : Lookup  InputValues=[0,0.1,0.2,0.3,0.4,0.5,0.6,0.7,0.8,1,2,3,4]  Table=[0,0,0.05,0.1,0.2,0.3,0.4,0.5,0.6,0.7,1,1,1]  SaturateOnIntegerOverflow=off
  Override : Gain  Gain=TV_Override
  Product : Product  RndMeth=Zero
  Read CM Dict : CarMaker4SL/Read CM Dict  xname=Car.muRoadFR  xsync=off  xstime=Continuous
  Read CM Dict1 : CarMaker4SL/Read CM Dict  xname=Car.v  xsync=off  xstime=Continuous
  Read CM Dict2 : CarMaker4SL/Read CM Dict  xname=Car.YawRate  xsync=off  xstime=Continuous
  Read CM Dict3 : CarMaker4SL/Read CM Dict  xname=VC.Steer.Ang  xsync=off  xstime=Continuous
  Subtract : Sum  Inputs=+-
  Switch : Switch  Criteria=u2 > Threshold  SaturateOnIntegerOverflow=off  InputSameDT=off
  TV FR : Outport  VectorParamsAs1DForOutWhenUnconnected=off
  wires:
  Read CM Dict/1 -> Gravity/1
  Gravity/1 -> Override/1
  Override/1 -> Divide/1
  Read CM Dict1/1 -> Switch/1, Switch/2
  Constant/1 -> Switch/3
  Switch/1 -> Abs/1
  Abs/1 -> Divide/2
  Divide/1 -> Subtract/1
  Read CM Dict2/1 -> Abs2/1
  Subtract/1 -> Product/1
  Product/1 -> TV FR/1
  Read CM Dict3/1 -> Gain/1
  Lookup Table/1 -> Product/2
  Abs2/1 -> Subtract/2
  Gain/1 -> Lookup Table/1

== system TorqueVect/CarMaker/IPG Vehicle/PowerTrain/PTControl Example/PTControl_TV_IPG/Torque Control 2/Electronic Gas Pedal RL ==
  TV_On : Inport
  VC.Gas : Inport  Port=2
  Define CM Dict : CarMaker4SL/Define CM Dict  xname=E_Gas_RL  xmono=off  xtype=Double4  xdvaplace=None  xnstates=0  xfirststate=0  xinitial=0
  Read CM Dict : CarMaker4SL/Read CM Dict  xname=E_Gas_RL  xsync=off  xstime=Continuous
  Read CM Dict1 : CarMaker4SL/Read CM Dict  xname=Car.LongSlipRL  xsync=off  xstime=Continuous
  Switch : Switch  Criteria=u2 > Threshold  SaturateOnIntegerOverflow=off  InputSameDT=off
  Traction Control RL : Subsystem
  Write CM Dict : CarMaker4SL/Write CM Dict  xname=E_Gas_RL  xsync=off
  Motor_Gas_RL : Outport  VectorParamsAs1DForOutWhenUnconnected=off
  wires:
  Traction Control RL/1(E_Gas) -> Write CM Dict/1, Switch/1
  TV_On/1 -> Switch/2
  Switch/1 -> Motor_Gas_RL/1
  VC.Gas/1 -> Traction Control RL/1(VC.Gas), Switch/3
  Read CM Dict1/1 -> Traction Control RL/3(Car.LongSlip)
  Read CM Dict/1 -> Traction Control RL/2(E_Gas.)

== system TorqueVect/CarMaker/IPG Vehicle/PowerTrain/PTControl Example/PTControl_TV_IPG/Torque Control 2/Torque Vectoring RL ==
  Abs : Abs  SaturateOnIntegerOverflow=off
  Abs2 : Abs  SaturateOnIntegerOverflow=off
  Constant : Constant
  Divide : Product  Inputs=*/
  Gain : Gain  Gain=-1
  Gravity : Gain  Gain=9.81
  Lookup Table : Lookup  InputValues=[0,0.1,0.2,0.3,0.4,0.5,0.6,0.7,0.8,1,2,3,4]  Table=[0,0,0.05,0.1,0.2,0.3,0.4,0.5,0.6,0.7,1,1,1]  SaturateOnIntegerOverflow=off
  Override : Gain  Gain=TV_Override
  Product : Product  RndMeth=Zero
  Read CM Dict : CarMaker4SL/Read CM Dict  xname=Car.muRoadRL  xsync=off  xstime=Continuous
  Read CM Dict1 : CarMaker4SL/Read CM Dict  xname=Car.v  xsync=off  xstime=Continuous
  Read CM Dict2 : CarMaker4SL/Read CM Dict  xname=Car.YawRate  xsync=off  xstime=Continuous
  Read CM Dict3 : CarMaker4SL/Read CM Dict  xname=VC.Steer.Ang  xsync=off  xstime=Continuous
  Subtract : Sum  Inputs=+-
  Switch : Switch  Criteria=u2 > Threshold  SaturateOnIntegerOverflow=off  InputSameDT=off
  TV RL : Outport  VectorParamsAs1DForOutWhenUnconnected=off
  wires:
  Read CM Dict/1 -> Gravity/1
  Gravity/1 -> Override/1
  Override/1 -> Divide/1
  Read CM Dict1/1 -> Switch/1, Switch/2
  Constant/1 -> Switch/3
  Switch/1 -> Abs/1
  Abs/1 -> Divide/2
  Divide/1 -> Subtract/1
  Read CM Dict2/1 -> Abs2/1
  Subtract/1 -> Product/1
  Product/1 -> TV RL/1
  Read CM Dict3/1 -> Gain/1
  Lookup Table/1 -> Product/2
  Abs2/1 -> Subtract/2
  Gain/1 -> Lookup Table/1

== system TorqueVect/CarMaker/IPG Vehicle/PowerTrain/PTControl Example/PTControl_TV_IPG/Torque Control 3/Electronic Gas Pedal RR ==
  TV_On : Inport
  VC.Gas : Inport  Port=2
  Define CM Dict : CarMaker4SL/Define CM Dict  xname=E_Gas_RR  xmono=off  xtype=Double4  xdvaplace=None  xnstates=0  xfirststate=0  xinitial=0
  Read CM Dict : CarMaker4SL/Read CM Dict  xname=E_Gas_RR  xsync=off  xstime=Continuous
  Read CM Dict1 : CarMaker4SL/Read CM Dict  xname=Car.LongSlipRR  xsync=off  xstime=Continuous
  Switch : Switch  Criteria=u2 > Threshold  SaturateOnIntegerOverflow=off  InputSameDT=off
  Traction Control RR : Subsystem
  Write CM Dict : CarMaker4SL/Write CM Dict  xname=E_Gas_RR  xsync=off
  Motor_Gas_RR : Outport  VectorParamsAs1DForOutWhenUnconnected=off
  wires:
  Read CM Dict/1 -> Traction Control RR/2(E_Gas.)
  Read CM Dict1/1 -> Traction Control RR/3(Car.LongSlip)
  VC.Gas/1 -> Switch/3, Traction Control RR/1(VC.Gas)
  Switch/1 -> Motor_Gas_RR/1
  TV_On/1 -> Switch/2
  Traction Control RR/1(E_Gas) -> Switch/1, Write CM Dict/1

== system TorqueVect/CarMaker/IPG Vehicle/PowerTrain/PTControl Example/PTControl_TV_IPG/Torque Control 3/Torque Vectoring RR ==
  Abs : Abs  SaturateOnIntegerOverflow=off
  Abs2 : Abs  SaturateOnIntegerOverflow=off
  Constant : Constant
  Divide : Product  Inputs=*/
  Gain : Gain  Gain=-1
  Gravity : Gain  Gain=9.81
  Lookup Table : Lookup  InputValues=[0,0.1,0.2,0.3,0.4,0.5,0.6,0.7,0.8,1,2,3,4]  Table=[0,0,0.05,0.1,0.2,0.3,0.4,0.5,0.6,0.7,1,1,1]  SaturateOnIntegerOverflow=off
  Override : Gain  Gain=TV_Override
  Product : Product  RndMeth=Zero
  Read CM Dict : CarMaker4SL/Read CM Dict  xname=Car.muRoadRR  xsync=off  xstime=Continuous
  Read CM Dict1 : CarMaker4SL/Read CM Dict  xname=Car.v  xsync=off  xstime=Continuous
  Read CM Dict2 : CarMaker4SL/Read CM Dict  xname=Car.YawRate  xsync=off  xstime=Continuous
  Read CM Dict3 : CarMaker4SL/Read CM Dict  xname=VC.Steer.Ang  xsync=off  xstime=Continuous
  Subtract : Sum  Inputs=+-
  Switch : Switch  Criteria=u2 > Threshold  SaturateOnIntegerOverflow=off  InputSameDT=off
  TV RR : Outport  VectorParamsAs1DForOutWhenUnconnected=off
  wires:
  Gain/1 -> Lookup Table/1
  Abs2/1 -> Subtract/2
  Lookup Table/1 -> Product/2
  Read CM Dict3/1 -> Gain/1
  Product/1 -> TV RR/1
  Subtract/1 -> Product/1
  Read CM Dict2/1 -> Abs2/1
  Divide/1 -> Subtract/1
  Abs/1 -> Divide/2
  Switch/1 -> Abs/1
  Constant/1 -> Switch/3
  Read CM Dict1/1 -> Switch/2, Switch/1
  Override/1 -> Divide/1
  Gravity/1 -> Override/1
  Read CM Dict/1 -> Gravity/1

== system TorqueVect/CarMaker/IPG Vehicle/PowerTrain/PTControl Example/PTControl_TV_MFE1/New TC/Reference Generator1 ==
  note: Modified slip ratio targets
  note: Vehicle velocity
  note: For throttle sign and Product:
      | If positive, normal reference
      | If negative (regen), similar reference but negative (negative target slip*times speed), this might need to change to account for regen limits
      | If 0, target zero
  x2 : Inport
  Front SR Target : Inport  Port=2
  Rear SR Target : Inport  Port=3
  Constant : Constant
  Product1 : Product
  Product2 : Product
  Switch : Switch  Criteria=u2 > Threshold  Threshold=1  SaturateOnIntegerOverflow=off  InputSameDT=off
  R1 : Outport
  L1 : Outport  Port=2
  R2 : Outport  Port=3
  L2 : Outport  Port=4
  wires:
  Front SR Target/1 -> Product1/1
  Product1/1 -> L1/1, R1/1
  Product2/1 -> L2/1, R2/1
  Rear SR Target/1 -> Product2/2
  Switch/1 -> Product2/1, Product1/2
  x2/1 -> Switch/1, Switch/2
  Constant/1 -> Switch/3
